simulink model "Ship_location_simulation_model_final"  (R2023b)
settings: Solver=VariableStepAuto  StartTime=0.0  StopTime=25  RelTol=1e-3
libraries: simulink x3
settings Model: Creator=Noy Kirshner  LastModifiedBy=Noy Kirshner

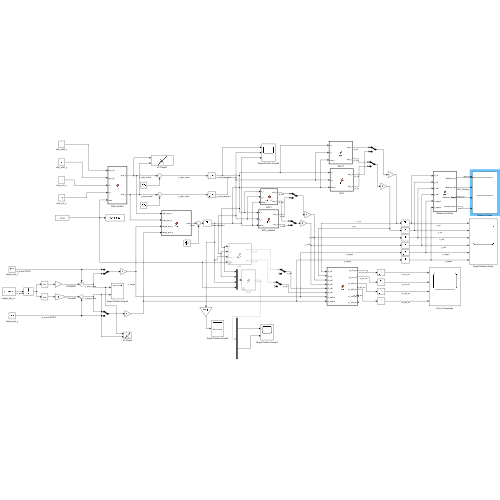
[thumbnail: Simulink's stored preview of the top-level diagram]
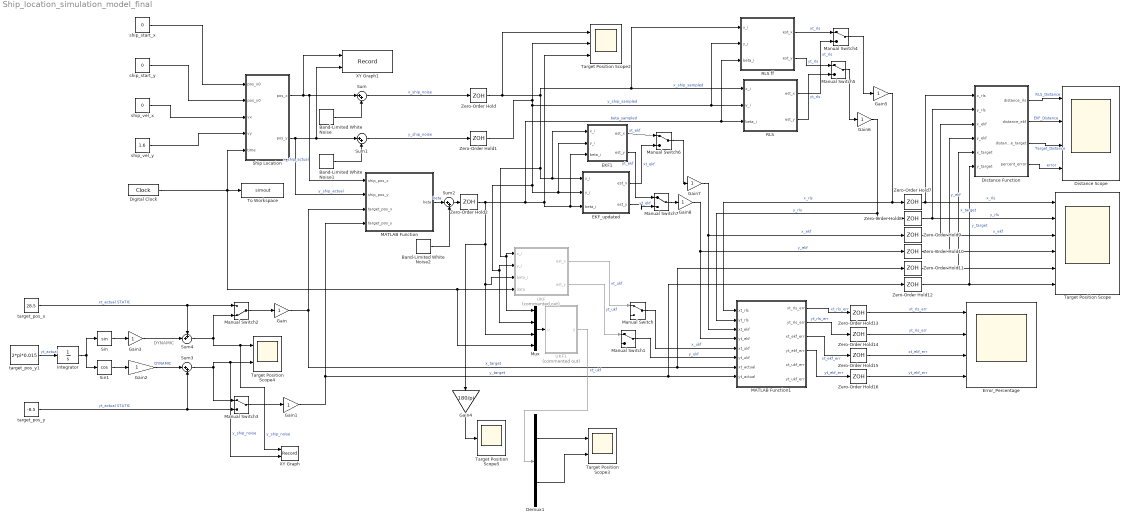
== system Ship_location_simulation_model_final ==
  note: DYNAMIC
  Band-Limited White Noise : simulink/Sources/Band-Limited White Noise  Cov=[0.01]  Ts=0.01  seed=[23341]
  Band-Limited White Noise1 : simulink/Sources/Band-Limited White Noise  Cov=[0.01]  Ts=0.01  seed=[233471]
  Band-Limited White Noise2 : simulink/Sources/Band-Limited White Noise  Cov=[0.000000001]  Ts=0.01  seed=[21113341]
  Demux1 : Demux  Outputs=2
  Digital Clock : DigitalClock  SampleTime=0.01
  Distance Function : MATLAB Function  TreatAsAtomicUnit=on
  Distance Scope : Scope  NumInputPorts=4
  EKF1 : MATLAB Function  TreatAsAtomicUnit=on
  EKF_updated : MATLAB Function  TreatAsAtomicUnit=on
  Error_Percentage : Scope  NumInputPorts=4
  Gain{,1..3,5..8} (8 alike) : Gain
  Gain4 : Gain  Gain=180/pi
  Integrator : Integrator
  MATLAB Function : MATLAB Function  TreatAsAtomicUnit=on
  MATLAB Function1 : MATLAB Function  TreatAsAtomicUnit=on
  Manual Switch{,1,3..7} (7 alike) : ManualSwitch
  Manual Switch2 : ManualSwitch  CurrentSetting=0
  Mux : Mux
  RLS : MATLAB Function  TreatAsAtomicUnit=on
  RLS ff : MATLAB Function  TreatAsAtomicUnit=on
  Ship Location : MATLAB Function  TreatAsAtomicUnit=on
  Sin : Trigonometry
  Sin1 : Trigonometry  Operator=cos
  Sum{,1..3} (4 alike) : Sum  Inputs=|++
  Sum4 : Sum  Inputs=++|
  Target Position Scope : Scope  NumInputPorts=6
  Target Position Scope2 : Scope  NumInputPorts=3
  Target Position Scope3 : Scope  NumInputPorts=2
  Target Position Scope4 : Scope  NumInputPorts=2
  Target Position Scope5 : Scope
  To Workspace : ToWorkspace  VariableName=simout  SaveFormat=Timeseries  SampleTime=-1
  UKF : MATLAB Function  Commented=on  TreatAsAtomicUnit=on
  UKF1 : MATLAB Function  Commented=on  TreatAsAtomicUnit=on
  XY Graph : Record  FileSettingsInternal="{\"entries\":[{\"content\":{\"excelSettings\":{\"content\":{},\"type\":\"Streamout.ExcelSettings\"}},\"type\":\"Streamout.FileSettingStorage\",\"uuid\":\"\"}],\"packageUris\":[\"http:\\/\\/schema.mathworks.com\\/mf0\\/streamout_blocks\\/R2020a\"],\"version\":\"1.0\"}"  Layout=[1 1]  SignalsInternal="{\"entries\":[{\"content\":{\"signals\":[{\"content\":{\"blockPath\":[],\"dimensions\":[1],\"domain\":\"\",\"lineColor\":\"#fe330a\",\"port\":1,\"sid\":[\"\"],\"signalID\":439,\"signalName\":\"y_ship_noise\"},\"type\":\"RecordBlkView.Signal\",\"uuid\":\"\"},{\"content\":{\"blockPath\":[],\"dimensions\":[1],\"domain\":\"\",\"lineColor\":\"#22b573\",\"port\":2,\"sid\":[\"\"],\"signalID\":443,\"signalName\":\"y_ship_noise\"},\"type\":\"RecordBlkView.Signal\",\"uuid\":\"\"}]},\"type\":\"RecordBlkView.InputSignals\",\"uuid\":\"\"}],\"packageUris\":[\"http:\\/\\/schema.mathworks.com\\/mf0\\/streamout_blocks\\/R2020a\"],\"version\":\"1.0\"}"  VisualizationBindings="{\"xyplotplugin\":{\"info\":[{\"series\":[],\"subplotID\":1}]}}"  CompatibilityTag=XY
  XY Graph1 : Record  FileSettingsInternal="{\"entries\":[{\"content\":{\"excelSettings\":{\"content\":{},\"type\":\"Streamout.ExcelSettings\"}},\"type\":\"Streamout.FileSettingStorage\",\"uuid\":\"\"}],\"packageUris\":[\"http:\\/\\/schema.mathworks.com\\/mf0\\/streamout_blocks\\/R2020a\"],\"version\":\"1.0\"}"  Layout=[1 1]  SignalsInternal="{\"entries\":[{\"content\":{\"signals\":[{\"content\":{\"blockPath\":[],\"dimensions\":[1],\"domain\":\"\",\"lineColor\":\"#0072bd\",\"port\":1,\"sid\":[\"\"],\"signalID\":447,\"signalName\":\"x_ship_actual\"},\"type\":\"RecordBlkView.Signal\",\"uuid\":\"\"},{\"content\":{\"blockPath\":[],\"dimensions\":[1],\"domain\":\"\",\"lineColor\":\"#d95319\",\"port\":2,\"sid\":[\"\"],\"signalID\":451,\"signalName\":\"y_ship_actual\"},\"type\":\"RecordBlkView.Signal\",\"uuid\":\"\"}]},\"type\":\"RecordBlkView.InputSignals\",\"uuid\":\"\"}],\"packageUris\":[\"http:\\/\\/schema.mathworks.com\\/mf0\\/streamout_blocks\\/R2020a\"],\"version\":\"1.0\"}"  VisualizationBindings="{\"xyplotplugin\":{\"info\":[{\"series\":[],\"subplotID\":1}]}}"  CompatibilityTag=XY
  Zero-Order Hold : ZeroOrderHold  SampleTime=0.01
  Zero-Order Hold1 : ZeroOrderHold  SampleTime=0.01
  Zero-Order Hold{7..16} (10 alike) : ZeroOrderHold
  Zero-Order Hold2 : ZeroOrderHold  SampleTime=0.01
  ship_start_x : Constant  Value=0
  ship_start_y : Constant  Value=0
  ship_vel_x : Constant  Value=0
  ship_vel_y : Constant  Value=1.6
  target_pos_x : Constant  Value=28.5
  target_pos_y : Constant  Value=-8.5
  target_pos_y1 : Constant  Value=2*pi*0.015
  wires:
  Digital Clock/1 -> Mux/4, UKF/4(data), Ship Location/5(time), To Workspace/1
  ship_start_x/1 -> Ship Location/1(pos_x0)
  ship_start_y/1 -> Ship Location/2(pos_y0)
  ship_vel_x/1 -> Ship Location/3(vx)
  ship_vel_y/1 -> Ship Location/4(vy)
  Ship Location/1(pos_x) -> XY Graph1/1, MATLAB Function/1(ship_pos_x), Sum/1  "x_ship_actual"
  Ship Location/2(pos_y) -> MATLAB Function/2(ship_pos_y), XY Graph1/2, Sum1/1  "y_ship_actual"
  Band-Limited White Noise/1 -> Sum/2
  Band-Limited White Noise1/1 -> Sum1/2
  target_pos_y/1 -> Sum3/2, Manual Switch3/2  "yt_actual STATIC"
  Band-Limited White Noise2/1 -> Sum2/2
  Sum1/1 -> Zero-Order Hold1/1  "y_ship_noise"
  Sum/1 -> Zero-Order Hold/1  "x_ship_noise"
  Sum2/1 -> Zero-Order Hold2/1
  MATLAB Function/1(beta) -> Sum2/1  "beta"
  MATLAB Function1/2(yt_rls_err) -> Zero-Order Hold14/1  "yt_rls_err"
  MATLAB Function1/1(xt_rls_err) -> Zero-Order Hold13/1  "xt_rls_err"
  MATLAB Function1/3(xt_ekf_err) -> Zero-Order Hold15/1  "xt_ekf_err"
  MATLAB Function1/4(yt_ekf_err) -> Zero-Order Hold16/1  "yt_ekf_err"
  Zero-Order Hold/1 -> Target Position Scope2/1, Mux/1, UKF/1(x_i), EKF1/1(x_i), EKF_updated/1(x_i), RLS ff/1(x_i), RLS/1(x_i)  "x_ship_sampled"
  Zero-Order Hold1/1 -> EKF1/2(y_i), EKF_updated/2(y_i), Mux/2, UKF/2(y_i), RLS ff/2(y_i), RLS/2(y_i), Target Position Scope2/2  "y_ship_sampled"
  Zero-Order Hold2/1 -> Target Position Scope2/3, EKF1/3(beta_i), EKF_updated/3(beta_i), RLS ff/3(beta_i), RLS/3(beta_i), Gain4/1, UKF/3(beta_i), Mux/3  "beta_sampled"
  RLS/1(est_x) -> Manual Switch4/2  "xt_rls"
  RLS/2(est_y) -> Manual Switch5/2  "yt_rls"
  UKF/1(est_x) -> Manual Switch/1  "xt_ukf"
  UKF/2(est_y) -> Manual Switch1/1  "yt_ukf"
  Manual Switch/1 -> MATLAB Function1/5(xt_ukf)  "x_ukf"
  Manual Switch1/1 -> MATLAB Function1/6(yt_ukf)  "y_ukf"
  Mux/1 -> UKF1/1(u)
  Demux1/1 -> Target Position Scope3/1
  Demux1/2 -> Target Position Scope3/2
  Gain/1 -> Zero-Order Hold11/1, MATLAB Function1/7(xt_actual), MATLAB Function/3(target_pos_x)  "x_target"
  Gain1/1 -> MATLAB Function/4(target_pos_y), Zero-Order Hold12/1, MATLAB Function1/8(yt_actual)  "y_target"
  target_pos_x/1 -> Manual Switch2/1, Sum4/1  "xt_actual STATIC"
  Manual Switch2/1 -> Gain/1
  Manual Switch3/1 -> Gain1/1
  Integrator/1 -> Sin/1, Sin1/1
  target_pos_y1/1 -> Integrator/1  "yt_actual"
  Sin1/1 -> Gain2/1
  Sin/1 -> Gain3/1
  Gain2/1 -> Sum3/1  "DYNAMIC"
  Gain3/1 -> Sum4/2
  Sum4/1 -> XY Graph/1, Target Position Scope4/1, Manual Switch2/2  "y_ship_noise"
  Sum3/1 -> Manual Switch3/1, XY Graph/2, Target Position Scope4/2  "y_ship_noise"
  Gain4/1 -> Target Position Scope5/1
  Gain5/1 -> MATLAB Function1/1(xt_rls), Zero-Order Hold7/1  "x_rls"
  Gain6/1 -> MATLAB Function1/2(yt_rls), Zero-Order Hold8/1  "y_rls"
  RLS ff/1(est_x) -> Manual Switch4/1  "xt_rls"
  RLS ff/2(est_y) -> Manual Switch5/1  "yt_rls"
  Manual Switch4/1 -> Gain5/1
  Manual Switch5/1 -> Gain6/1
  Gain7/1 -> Zero-Order Hold9/1, MATLAB Function1/3(xt_ekf)  "x_ekf"
  Gain8/1 -> Zero-Order Hold10/1, MATLAB Function1/4(yt_ekf)  "y_ekf"
  EKF1/1(est_x) -> Manual Switch6/1  "xt_ekf"
  EKF_updated/1(est_x) -> Manual Switch6/2  "xt_ekf"
  Manual Switch6/1 -> Gain7/1
  Manual Switch7/1 -> Gain8/1
  EKF_updated/2(est_y) -> Manual Switch7/2  "yt_ekf"
  EKF1/2(est_y) -> Manual Switch7/1  "yt_ekf"
  UKF1/1(y) -> Demux1/1  "xt_ukf"
  Zero-Order Hold7/1 -> Distance Function/1(x_rls), Target Position Scope/1  "x_rls"
  Zero-Order Hold8/1 -> Distance Function/2(y_rls), Target Position Scope/2  "y_rls"
  Zero-Order Hold9/1 -> Distance Function/3(x_ekf), Target Position Scope/3  "x_ekf"
  Zero-Order Hold10/1 -> Distance Function/4(y_ekf), Target Position Scope/4  "y_ekf"
  Zero-Order Hold11/1 -> Distance Function/5(x_target), Target Position Scope/5  "x_target"
  Zero-Order Hold12/1 -> Distance Function/6(y_target), Target Position Scope/6  "y_target"
  Zero-Order Hold13/1 -> Error_Percentage/1  "xt_rls_err"
  Zero-Order Hold14/1 -> Error_Percentage/2  "yt_rls_err"
  Zero-Order Hold15/1 -> Error_Percentage/3  "xt_ekf_err"
  Zero-Order Hold16/1 -> Error_Percentage/4  "yt_ekf_err"
  Distance Function/2(distance_ekf) -> Distance Scope/2  "EKF_Distance"
  Distance Function/3(distance_target) -> Distance Scope/3  "Target_Distance"
  Distance Function/1(distance_rls) -> Distance Scope/1  "RLS_Distance"
  Distance Function/4(percent_error) -> Distance Scope/4  "error"

== matlab function Ship_location_simulation_model_final/EKF1 ==
  data: x_i input; est_x output; y_i input; beta_i input; est_y output
function [est_x, est_y] = ekf_fcn(x_i, y_i, beta_i)

persistent X_i P Q R

if isempty(P)
    P = 1000000*eye(6); % Covariance matrix initialization (6x6)
    Q = 0.1*diag([0.01, 0.01, 1, 0.01, 1, 0.01]); % Process noise covariance initialization (6x6)
    R = diag([1, 1, 100000]); % Measurement noise covariance initialization (3x3)
end

if isempty(X_i)
    X_i = zeros(6, 1); % State vector initialization (6x1)
end

dt = 0.01; % Sample time variable
F = [1 0 0 0 0 0 ; 0 1 0 0 0 0 ; 0 0 1 dt 0 0 ; 0 0 0 1 0 0 ; 0 0 0 0 1 dt ; 0 0 0 0 0 1]; % Process Jacobian (6x6)
H = [0 0 1 0 0 0 ; 0 0 0 0 1 0 ; sin(beta_i) -cos(beta_i) -sin(beta_i) 0 cos(beta_i) 0]; % Measurement Jacobian (3x6)

% Prediction Step
X_i = F*X_i; % Process Model
meas = [x_i ; y_i ; 0]; % Measurements
y_hat = H*X_i; % Measurement Model
P = F*P*F' + Q; % Covariance matrix

% Update Step
resid = meas - y_hat; % Measurement residual
K = P*H'/(H*P*H' + R); % Kalman gain
X_i = X_i + K*resid; % State vector update
P = (eye(6) - K*H)*P; % Covariance matrix update

% Output estimated position
est_x = X_i(1); % x_t estimation
est_y = X_i(2); % y_t estimation

end

== matlab function Ship_location_simulation_model_final/Distance Function ==
  data: x_rls input; distance_rls output; y_rls input; x_ekf input; y_ekf input; distance_ekf output; x_target input; y_target input; distance_target output; percent_error output
function [distance_rls,distance_ekf,distance_target,percent_error]= fcn(x_rls,y_rls,x_ekf,y_ekf,x_target,y_target)

distance_rls = sqrt(x_rls^2 + y_rls^2);
distance_ekf = sqrt(x_ekf^2 + y_ekf^2);
distance_target = sqrt(x_target^2 + y_target^2);
percent_error = 0.9*distance_target;

== matlab function Ship_location_simulation_model_final/MATLAB Function ==
  data: ship_pos_x input; beta output; ship_pos_y input; target_pos_x input; target_pos_y input
function beta = fcn(ship_pos_x,ship_pos_y,target_pos_x,target_pos_y)

dx = target_pos_x - ship_pos_x;
dy = target_pos_y - ship_pos_y;

beta = atan2(dy,dx);

== matlab function Ship_location_simulation_model_final/Ship Location ==
  data: pos_x0 input; pos_x output; pos_y0 input; vx input; vy input; time input; pos_y output
function [pos_x,pos_y] = fcn(pos_x0,pos_y0,vx,vy,time)

pos_x = vx*time + pos_x0;
pos_y = vy*time + pos_y0;

== matlab function Ship_location_simulation_model_final/RLS ==
  data: x_i input; est_x output; y_i input; beta_i input; est_y output
function [est_x, est_y] = fcn(x_i, y_i, beta_i)

persistent P X_i
gamma=0.55;
if isempty(P)
    P = eye(2);  % Covariance matrix initialization
end

if isempty(X_i)
    X_i = zeros(2, 1);  % X vector initialization as a zero vector
end

phi_i = [-sin(beta_i); cos(beta_i)]; % Update phi vector
z_i = y_i * cos(beta_i) - x_i * sin(beta_i); % z_i 
e = z_i - phi_i' * X_i; % update error vector
X_i = X_i + P * phi_i / (gamma + phi_i' * P * phi_i) * e; % Update X vector

g_k = P * phi_i / (1 + phi_i' * P * phi_i); % Weight vector
P = P - g_k * phi_i' * P; % Covariance matrix update

% Update estimated position
est_x = X_i(1);
est_y = X_i(2);

end

== matlab function Ship_location_simulation_model_final/MATLAB Function1 ==
  data: xt_rls input; xt_rls_err output; yt_rls input; xt_ekf input; yt_ekf input; xt_ukf input; yt_ukf input; xt_actual input; yt_actual input; yt_rls_err output; xt_ekf_err output; yt_ekf_err output; xt_ukf_err output; yt_ukf_err output
function [xt_rls_err,yt_rls_err,xt_ekf_err,yt_ekf_err,xt_ukf_err,yt_ukf_err] = fcn(xt_rls,yt_rls,xt_ekf,yt_ekf,xt_ukf,yt_ukf, xt_actual,yt_actual)

% RLS error values:
xt_rls_err = ((xt_rls - xt_actual)/xt_actual)*100;
yt_rls_err = ((yt_rls - yt_actual)/yt_actual)*100;

% EKF error values:
xt_ekf_err = ((xt_ekf - xt_actual)/xt_actual)*100;
yt_ekf_err = ((yt_ekf - yt_actual)/yt_actual)*100;

% UKF error values:
xt_ukf_err = 0;
yt_ukf_err = 0;
%xt_ukf_err = (abs(xt_ukf - xt_actual)/xt_actual)*100;
%yt_ukf_err = (abs(yt_ukf - yt_actual)/yt_actual)*100;

== matlab function Ship_location_simulation_model_final/EKF_updated ==
  data: x_i input; est_x output; y_i input; beta_i input; est_y output
function [est_x, est_y] = ekf_fcn(x_i, y_i, beta_i)

persistent X_i P Q R

if isempty(P)
    P = 1000000000*eye(8); % Covariance matrix initialization (8x8)
    Q = 10000*diag([1, 0.01, 1, 0.01, 1, 0.01, 1, 0.01]); % Process noise covariance initialization (8x8)
    R = diag([10, 10, 40000000]); % Measurement noise covariance initialization (3x3)
end
 
if isempty(X_i)
    X_i = zeros(8, 1); % State vector initialization (8x1)
end

dt = 0.001; % Sample time variable
F = [1 dt 0 0 0 0 0 0 ; 0 1 0 0 0 0 0 0 ; 0 0 1 dt 0 0 0 0 ; 0 0 0 1 0 0 0 0 ; 0 0 0 0 1 dt 0 0 ; 0 0 0 0 0 1 0 0 ; 0 0 0 0 0 0 1 dt ; 0 0 0 0 0 0 0 1]; % Process Jacobian (8x8)
H = [0 0 0 0 1 0 0 0 ; 0 0 0 0 0 0 1 0 ; sin(beta_i) 0 -cos(beta_i) 0 -sin(beta_i) 0 cos(beta_i) 0]; % Measurement Jacobian (3x8)

% Prediction Step
X_i = F*X_i; % Process Model
meas = [x_i ; y_i ; 0]; % Measurements
y_hat = H*X_i; % Measurement Model
P = F*P*F' + Q; % Covariance matrix

% Update Step
resid = meas - y_hat; % Measurement residual
K = P*H'/(H*P*H' + R); % Kalman gain
X_i = X_i + K*resid; % State vector update
P = (eye(8) - K*H)*P; % Covariance matrix update

% Output estimated position
est_x = X_i(1); % x_t estimation
est_y = X_i(3); % y_t estimation

end

== matlab function Ship_location_simulation_model_final/UKF ==
  data: x_i input; est_x output; y_i input; beta_i input; est_y output; data input
function [est_x, est_y] = ukf_fcn(x_i, y_i, beta_i, data)
    persistent X_i Px_pred Pz Pxz Q R C Wm Wc
    
    a = 10^-3;
    b = 2;
    k = 0;
    lambda = a^2 * (6 + k) - 6;

           C = [0 0 1 0 0 0;
             0 0 0 0 1 0;
             sin(beta_i) -cos(beta_i) -sin(beta_i) 0 cos(beta_i) 0];
    
   % if isempty(X_i)
Px_pred = 1000000 * eye(6);
 X_i = ones(6, 1);
  Q = 0.1 * diag([0.01, 0.01, 1, 0.01, 1, 0.01]);
   if data<0.1
        % Initialize state vector (6x1)
        X_i = ones(6, 1);

        % Initialize state covariance matrix (6x6)
        Px_pred = 1000000 * eye(6);

        % Initialize measurement covariance matrix (3x3)
        Pz = zeros(3,3);

        % Initialize measurement covariance matrix (3x3)
        Pxz = zeros(6,3);

        % Process noise covariance (6x6)
        Q = 0.1 * diag([0.01, 0.01, 1, 0.01, 1, 0.01]);

        % Measurement noise covariance (3x3)
        R = diag([1, 1, 100000]);

        % Measurement matrix (3x6)
        C = [0 0 1 0 0 0;
             0 0 0 0 1 0;
             sin(beta_i) -cos(beta_i) -sin(beta_i) 0 cos(beta_i) 0];
   else
 
    % UKF weights initialization
    L = length(X_i);
    gamma = sqrt(lambda + L);
    
    if isempty(Wm)
        Wm = zeros(2 * L + 1, 1);
        Wc = zeros(2 * L + 1, 1);
        Wm(1) = lambda / (gamma^2);
        Wc(1) = Wm(1) + (1 - a^2 + b);
        for i = 2:2 * L + 1
            Wm(i) = 1 / (2 * gamma^2);
            Wc(i) = Wm(i);
        end
    end

    % Prediction Step
    % Generate sigma points
    S = chol(Px_pred)';
    X = [zeros(size(X_i)) S -S];
    X = gamma * X + repmat(X_i, 1, size(X, 2));
    x_pred = X * Wm;

    % Predicted state covariance
    for i = 1 : 2 * L + 1
        
   dt = 0.01; % Sample time variable
           F = [1 0 0 0 0 0 ; 0 1 0 0 0 0 ; 0 0 1 dt 0 0 ; 0 0 0 1 0 0 ; 0 0 0 0 1 dt ; 0 0 0 0 0 1]; % Process Jacobian (6x6)Px_pred = Px_pred + Wc(i) * (X - x_pred) * (X - x_pred)';
    end

    Px_pred = F*Px_pred*F' + Q;

    % Update Step
    % Generate sigma points
    S = chol(Px_pred)';
    X = [zeros(size(X_i)) S -S];
    X = gamma * X + repmat(x_pred, 1, size(X, 2));

    % Predicted measurements
    Z = C * X;
    z_pred = Z * Wm;

    % Measurement covariance
    for i = 1 : 2 * L + 1
        Pz = Pz + Wc(i) * (Z - z_pred) * (Z - z_pred)';
    end
    Pz = Pz + R;

    % Cross-covariance
    for i = 1 : 2 * L + 1
        Pxz = Pxz + Wc(i) * (X - repmat(x_pred, 1, size(X, 2))) * (Z - repmat(z_pred, 1, size(Z, 2)))';
    end
    
    % Kalman gain
    K = Pxz / Pz;

    % Residual (measurement error)
    meas = [x_i; y_i; 0]; % Assuming z-measurement is [x_i; y_i; 0]
    resid = meas - z_pred;

    % Update state estimate
    X_i = x_pred + K * resid;

    % Update state covariance
    Px_pred = abs(Px_pred - K * Pz * K');
    
    % Estimated position
    est_x = X_i(1);
    est_y = X_i(2);
    
   end
end

== matlab function Ship_location_simulation_model_final/UKF1 ==
  data: u input; y output
%function [est_x, est_y] = ukf_fcn(x_i, y_i, beta_i, data)
function y = fcn(u)

   persistent X_i ;
   if isempty (X_i)
     X_i  = ones(6, 1);     
   end
   
   persistent   ex ;
   if isempty (ex)
     ex = ones(3, 1);     
   end  

 



      persistent Xa ;
   if isempty (Xa)
     Xa  = ones(6, 6);     
   end
 
      persistent Xb ;
   if isempty (Xb)
     Xb  = zeros(6, 12);     
   end



      persistent Z ;
   if isempty (Z)
     Z  = zeros(3, 12);     
   end
   
      persistent Pz
      if isempty (Pz)
     Pz  = ones(3, 3);     
      end


      persistent Pxz
      if isempty (Pxz)
     Pxz  = zeros(6, 3);     
      end


   persistent Px_pred ; 
   if isempty(Px_pred)  
     Px_pred = 1000000 * eye(6);
   end


   persistent S ; 
   if isempty(S)  
     S = 1000000 * eye(6);
   end





   persistent x_pred ; 
   if isempty(x_pred)  
     x_pred =  zeros(6,1);
   end


   persistent z_pred ; 
   if isempty(z_pred)  
     z_pred =  zeros(3,1);
   end

  persistent z_predd ; 
   if isempty(z_predd)  
     z_predd =  zeros(3,12);
   end



   persistent x_predd ; 
   if isempty(x_predd)  
     x_predd =  zeros(6,12);
   end



   persistent F; 
   if isempty(F)
 F = [1 0 0 0 0 0 ; 0 1 0 0 0 0 ; 0 0 1 0.01 0 0 ; 0 0 0 1 0 0 ; 0 0 0 0 1 0.01 ; 0 0 0 0 0 1];
   end 
 
  
 persistent Q ;
 if isempty(Q)
 Q =  10*diag([0.01, 0.01, 1, 0.01, 1, 0.01]);
 end


 persistent R;
 if isempty(R)
  R = diag([1, 10 , 100 ]);
 end
 
 persistent   C  ;
  if isempty(C)
        C = [0 0 1 0 0 0;
             0 0 0 0 1 0;
             sin(u(3)) -cos(u(3)) -sin(u(3)) 0 cos(u(3)) 0];
  end

 

 
    if u(4)<0.05

   dt = 0.01; % Sample time variable
           F = [1 0 0 0 0 0 ; 0 1 0 0 0 0 ; 0 0 1 dt 0 0 ; 0 0 0 1 0 0 ; 0 0 0 0 1 dt ; 0 0 0 0 0 1]; % Process Jacobian (6x6)
         %         % Process noise covariance (6x6)
         Q =   1*diag([1, 1, 0.1,  1, 0.1,  1]);

%         % Initialize state vector (6x1)
         x_pred = zeros(6, 1);
           x_pred(1,1)=30;
         x_pred(2,1)=30;
%         x_pred(3,1)=-0.5;
% 
%         % Initialize state covariance matrix (6x6)
        %  Px_pred = 1000000*eye(6);
    
      S = (chol(Px_pred));
              Xa=repmat(x_pred, 1, 6);   
              X = [ (((6)^0.5))*(S)+Xa  , (((6)^0.5))*(-S)+Xa];
               Xb=F*X;
             
              

                   x_pred = (1/12)*(sum(Xb,2)); 
            
                   x_predd = repmat(x_pred, 1, 12); 

    % Predicted state covariance
 
                                   
          Px_pred = (1/12)*(Xb - x_predd) * (Xb - x_predd)';
        %   Px_pred = F*Px_pred*F'+ Q;
% 
% 
% 

% 
%         % Measurement noise covariance (3x3)
         R =       0.01*diag([5, 5, 1000 ]);
% 
%         % Measurement matrix (3x6)
            C = [0 0 1 0 0 0;
                0 0 0 0 1 0;
                 1*sin(u(3))  -cos(u(3))*1  -sin(u(3))*1  0 cos(u(3))*1  0];
% 
        
         % y=zeros(2,1);
    end
 
 
    

       S = (chol(Px_pred));
    Xa=repmat(x_pred, 1, 6);
   
    X =  [   ((6)^0.5)*(S)+Xa  , (((6)^0.5))*(-S)+Xa ];
   
       
    Xb=F*X;
   

     x_pred = (1/12)*(sum(Xb,2)); 
     x_predd = repmat(x_pred, 1, 12); 
 
    % Predicted state covariance
 
        Px_pred =   (1/12)*(Xb - x_predd) * (Xb - x_predd)' ;
        Px_pred =    Px_pred  +Q;


   %  Z=C*Xb;
%
        for j=1,12;
%          
             Z(1,j)=Xb(3,j);
              Z(2,j)=Xb(5,j);
              Z(3,j)=atan2(Xb(2,j)-Xb(5,j),Xb(1,j)-Xb(3,j));
            %  Z(3,j)=atan((Xb(2,j)-Xb(5,j))/(Xb(1,j)-Xb(3,j)));
%          
         end

   
    z_pred =(1/12)*sum(Z,2) ;
    z_predd=repmat( z_pred, 1, 12);   
    
    
    % Measurement covariance
 
        Pz = (1/12)*(Z - z_predd) * (Z - z_predd)'+R;
  

    % Cross-covariance
 
        Pxz = (1/12)*(Xb - (x_predd)) * (Z - (z_predd))';
   
    
    % Kalman gain
    K = Pxz/(Pz);

    % Residual (measurement error)
    meas = [u(1); u(2); 1*u(3)];  
    ex = meas - z_pred;

    % Update state estimate
   x_pred = x_pred + K * (ex);

    % Update state covariance
    Px_pred = Px_pred - K * Pz * K';
    
   % f1=atan2((x_pred(2,1)-x_pred(5,1)),(x_pred(1,1)-x_pred(3,1)));

    %   y=[ z_pred(1,1),u(1), z_pred(2,1),u(2), z_pred(3,1),u(3), f1,x_pred(2,1)];

   %     y=[ x_pred(1,1),  x_pred(2,1),u(2), z_pred(3,1),u(3), f1,x_pred(2,1)];
     %   y=[ z_pred(1,1),u(1), z_pred(2,1),u(2), z_pred(3,1),u(3)   ];
  
% y=[   ex(3,1),ex(2,1)   ];

  y=[   z_pred(3,1),u(3)   ];

%   y=[   x_pred(1,1),  x_pred(2,1)  ];

== matlab function Ship_location_simulation_model_final/RLS ff ==
  data: x_i input; est_x output; y_i input; beta_i input; est_y output
function [est_x, est_y] = fcn(x_i, y_i, beta_i)

persistent P X_i lambda lambda_o

if isempty(P)
    P = eye(2);  % Covariance matrix initialization
    lambda_o = 0.8;
    lambda = 0.5;
end

if isempty(X_i)
    X_i = zeros(2, 1);  % X vector initialization as a zero vector
end


phi_i = [-sin(beta_i); cos(beta_i)]; % Update phi vector
z_i = y_i * cos(beta_i) - x_i * sin(beta_i); % z_i 
e = z_i - phi_i' * X_i; % update error vector
X_i = X_i + P * phi_i / (lambda + phi_i' * P * phi_i) * e; % Update X vector

g_k = P * phi_i / (lambda + phi_i' * P * phi_i); % Weight vector
P = (1 / lambda)* (P - g_k * phi_i' * P); % Covariance matrix update with forgetting factor
lambda = lambda_o*lambda + (1 -lambda_o);

% Update estimated position
est_x = X_i(1);
est_y = X_i(2);

end
